simulink model "aaaqi"  (R2016b)
settings: Solver=ode4  StartTime=0.0  StopTime=inf  FixedStep=0.002  RelTol=1e-3  EnableMultiTasking=on
undefined symbols (not defined in the file or in its folder): bit, mdaadlink6208, sigbuilder_block, Standard
libraries: slrtlib x20, slrtsoftinglib x11, simulink x10
(part 2 of 4)

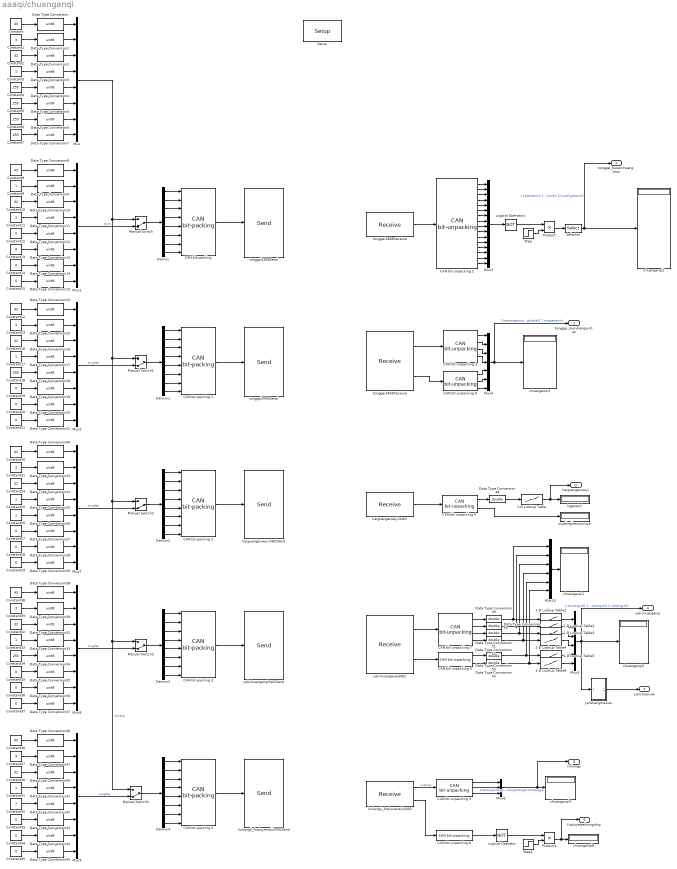
== system aaaqi/chuanganqi ==
  1-D Lookup Table : Lookup_n-D  NumberOfTableDimensions=1  BreakpointsForDimension1=[80 8500]  Table=[0 600]  InternalRulePriority=Speed  RndMeth=Simplest  InputSameDT=on
  1-D Lookup Table1 : Lookup_n-D  NumberOfTableDimensions=1  BreakpointsForDimension1=[1022 6022]  Table=[0 0.5]  InternalRulePriority=Speed  RndMeth=Simplest  InputSameDT=on
  1-D Lookup Table2 : Lookup_n-D  NumberOfTableDimensions=1  BreakpointsForDimension1=[1024 6018]  Table=[0 0.5]  InternalRulePriority=Speed  RndMeth=Simplest  InputSameDT=on
  1-D Lookup Table3 : Lookup_n-D  NumberOfTableDimensions=1  BreakpointsForDimension1=[999 5991]  Table=[0 0.5]  InternalRulePriority=Speed  RndMeth=Simplest  InputSameDT=on
  1-D Lookup Table4 : Lookup_n-D  NumberOfTableDimensions=1  BreakpointsForDimension1=[1006 6005]  Table=[0 0.5]  InternalRulePriority=Speed  RndMeth=Simplest  InputSameDT=on
  1-D Lookup Table5 : Lookup_n-D  NumberOfTableDimensions=1  BreakpointsForDimension1=[1010 6012]  Table=[0 0.5]  InternalRulePriority=Speed  RndMeth=Simplest  InputSameDT=on
  1-D Lookup Table6 : Lookup_n-D  NumberOfTableDimensions=1  BreakpointsForDimension1=[1024 6020]  Table=[0 0.5]  InternalRulePriority=Speed  RndMeth=Simplest  InputSameDT=on
  CAN bit-packing {,1..4} (5 alike) : slrtlib/CAN/Utilities/CAN bit-packing   bitpatterns={ [0:7] [8:15] [16:23] [24:31] [32:39] [40:47] [48:55] [56:63]}
  CAN bit-unpacking 2 : slrtlib/CAN/Utilities/CAN bit-unpacking   bitpatterns={0 1 2 3 4 5 6 7 8 9 10 11 12 13 14 15}  dtypes={ 'boolean','boolean','boolean','boolean','boolean','boolean','boolean','boolean','boolean','boolean','boolean','boolean','boolean','boolean','boolean','boolean'}
  CAN bit-unpacking 3 : slrtlib/CAN/Utilities/CAN bit-unpacking   bitpatterns={ [0:15],[16:31],[32:47],[48:63]}  dtypes={ 'uint16','uint16','uint16','uint16' }
  CAN bit-unpacking 4 : slrtlib/CAN/Utilities/CAN bit-unpacking   bitpatterns={ [0:15],[16:31]}  dtypes={ 'uint16','uint16'}
  CAN bit-unpacking 5 : slrtlib/CAN/Utilities/CAN bit-unpacking   bitpatterns={ [0:15] [16:31] [32:47]}  dtypes={ 'uint16','uint16','uint16'}
  CAN bit-unpacking 6 : slrtlib/CAN/Utilities/CAN bit-unpacking   bitpatterns={ [0:15],[16:31]}  dtypes={'uint16','uint16' }
  CAN bit-unpacking 7 : slrtlib/CAN/Utilities/CAN bit-unpacking   bitpatterns={ [0:15],[16:31],[32:47],[48:63]}  dtypes={ 'uint16','uint16','uint16','uint16' }
  CAN bit-unpacking 8 : slrtlib/CAN/Utilities/CAN bit-unpacking   bitpatterns={0}  dtypes={ 'boolean'}
  CAN bit-unpacking 9 : slrtlib/CAN/Utilities/CAN bit-unpacking   bitpatterns={ [0:15],[16:31],[32:47]}  dtypes={'uint16','uint16','uint16' }
  Constant{,8,22,30,38,46} (6 alike) : Constant  Value=43
  Constant{1,23,31,39,47} (5 alike) : Constant  Value=3
  Constant{2,10,16,24,32,40} (6 alike) : Constant  Value=32
  Constant{3,9,11,17,25..26,33,41} (8 alike) : Constant
  Constant{12..15,19..21,27..29,35..37,43..45} (16 alike) : Constant  Value=0
  Constant{4..7,18,34} (6 alike) : Constant  Value=255
  Constant42 : Constant  Value=7
  Data Type Conversion{,1..47} (48 alike) : DataTypeConversion  OutDataTypeStr=uint8
  Data Type Conversion{48..54} (7 alike) : DataTypeConversion  OutDataTypeStr=double
  Demux{,1..4} (5 alike) : Demux  Outputs=8
  Logical Operator : Logic  Operator=NOT  AllPortsSameDT=off  OutDataTypeStr=boolean
  Logical Operator1 : Logic  Operator=NOT  AllPortsSameDT=off  OutDataTypeStr=boolean
  Manual Switch{,1..4} (5 alike) : ManualSwitch  CurrentSetting=0
  Mux{,1..2,7..9} (6 alike) : Mux  Inputs=8
  Mux10 : Mux  Inputs=6
  Mux3 : Mux  Inputs=16
  Mux4 : Mux  Inputs=7
  Mux5 : Mux  Inputs=6
  Mux6 : Mux  Inputs=3
  Product : Product
  Product1 : Product
  Selector : Selector  IndexOptions=Index vector (dialog)  Indices=[5:16]  OutputSizes=[(-2)]
  "Setup " : slrtsoftinglib/CAN-AC2-PCI SJA 1000/Setup   board=1  can1bus=Highspeed (ISO 11898)  can1Baudrate=1 MBaud  can1UserBR=[1,1,4,3]  can2bus=Highspeed (ISO 11898)  can2Baudrate=500 kBaud  can2UserBR=[1,1,4,3]  init=[]  term=[]  bus_off_out=off  bus_off_rec=Off  ioBaseAddress=-1
  Step : Step  Time=0.2  SampleTime=0
  Step1 : Step  Time=0.2  SampleTime=0
  chuanganqi{1..5,8} (6 alike) : Display
  kaiguangaiweiyi3402 : slrtsoftinglib/CAN-AC2-PCI SJA 1000/Receive   board=1  canPort=CAN 1  range=Standard (11-bit)  ids=387  lengths=8  output=Data  inten=off  ts=-1  ididx=[2]
  kaiguangaiweiyi3402Send : slrtsoftinglib/CAN-AC2-PCI SJA 1000/Send   board=1  canPort=CAN 2  range=Standard (11-bit)  ids=1539  sizes=[8]  output=off  ts=-1  ididx=[1]
  kggweiyi : Display
  liuliangji_fuqiuyeweiji3402 : slrtsoftinglib/CAN-AC2-PCI SJA 1000/Receive   board=1  canPort=CAN 1  range=Standard (11-bit)  ids=[389 1157]  lengths=8  output=Data  inten=off  ts=-1  ididx=[4,7]
  liuliangji_fuqiuyeweiji3402Send : slrtsoftinglib/CAN-AC2-PCI SJA 1000/Send   board=1  canPort=CAN 2  range=Standard (11-bit)  ids=1541  sizes=[8]  output=off  ts=-1  ididx=[3]
  suodingjiesuoyouya : Display
  tonggai1808Receive : slrtsoftinglib/CAN-AC2-PCI SJA 1000/Receive   board=1  canPort=CAN 1  range=Standard (11-bit)  ids=385  lengths=8  output=Data  inten=off  ts=-1  ididx=[0]
  tonggai1808Send : slrtsoftinglib/CAN-AC2-PCI SJA 1000/Send   board=1  canPort=CAN 1  range=Standard (11-bit)  ids=1537  sizes=[8]  output=off  ts=-1  ididx=[0]
  tonggai3402Receive : slrtsoftinglib/CAN-AC2-PCI SJA 1000/Receive   board=1  canPort=CAN 1  range=Standard (11-bit)  ids=[386 642]  lengths=8  output=Data  inten=off  ts=-1  ididx=[1,5]
  tonggai3402Send : slrtsoftinglib/CAN-AC2-PCI SJA 1000/Send   board=1  canPort=CAN 2  range=Standard (11-bit)  ids=1538  sizes=[8]  output=off  ts=-1  ididx=[0]
  yalichuanganqi3402 : slrtsoftinglib/CAN-AC2-PCI SJA 1000/Receive   board=1  canPort=CAN 1  range=Standard (11-bit)  ids=[388 644]  lengths=8  output=Data  inten=off  ts=-1  ididx=[3,6]
  yalichuanganqi3402Send : slrtsoftinglib/CAN-AC2-PCI SJA 1000/Send   board=1  canPort=CAN 2  range=Standard (11-bit)  ids=1540  sizes=[8]  output=off  ts=-1  ididx=[2]
  yalishangxiaxian : Subsystem
  tonggai_huoerchuanganqi : Outport
  tonggai_moniliangxinhao : Outport  Port=2
  kaiguangaiweiyi : Outport  Port=3
  yalichuanganqi : Outport  Port=4
  liuliangji : Outport  Port=5
  fuqiuyeweikongzhiqi : Outport  Port=6
  yalichaoxian : Outport  Port=7
  wires:
  CAN bit-unpacking 3/1 -> Mux4/1
  CAN bit-unpacking 3/2 -> Mux4/2
  CAN bit-unpacking 3/3 -> Mux4/3
  CAN bit-unpacking 3/4 -> Mux4/4
  CAN bit-unpacking 4/1 -> Data Type Conversion48/1
  Mux3/1 -> Logical Operator1/1
  Mux4/1 -> tonggai_moniliangxinhao/1, chuanganqi3/1  "1.kaiguangaiyouya1 2.kaiguangaiyouya2 3.xuansongjinweiyi1 4.xuansongjinweiyi2 5.xuansongjinlayali1 6.xuansongjinlayali2 7.tonggaijiasudu"
  kaiguangaiweiyi3402/1 -> CAN bit-unpacking 4/1
  tonggai3402Receive/1 -> CAN bit-unpacking 3/1
  tonggai1808Receive/1 -> CAN bit-unpacking 2/1
  Data Type Conversion/1 -> Mux/1
  Data Type Conversion1/1 -> Mux/2
  Data Type Conversion2/1 -> Mux/3
  Data Type Conversion3/1 -> Mux/4
  Data Type Conversion4/1 -> Mux/5
  Data Type Conversion5/1 -> Mux/6
  Data Type Conversion6/1 -> Mux/7
  Data Type Conversion7/1 -> Mux/8
  Demux/1 -> "CAN bit-packing "/1
  Demux/2 -> "CAN bit-packing "/2
  Demux/3 -> "CAN bit-packing "/3
  Demux/4 -> "CAN bit-packing "/4
  Demux/5 -> "CAN bit-packing "/5
  Demux/6 -> "CAN bit-packing "/6
  Demux/7 -> "CAN bit-packing "/7
  Demux/8 -> "CAN bit-packing "/8
  "CAN bit-packing "/1 -> tonggai1808Send/1
  Constant/1 -> Data Type Conversion/1
  Constant1/1 -> Data Type Conversion1/1
  Constant2/1 -> Data Type Conversion2/1
  Constant3/1 -> Data Type Conversion3/1
  Constant4/1 -> Data Type Conversion4/1
  Constant5/1 -> Data Type Conversion5/1
  Constant6/1 -> Data Type Conversion6/1
  Constant7/1 -> Data Type Conversion7/1
  Demux1/1 -> CAN bit-packing 1/1
  Demux1/2 -> CAN bit-packing 1/2
  Demux1/3 -> CAN bit-packing 1/3
  Demux1/4 -> CAN bit-packing 1/4
  Demux1/5 -> CAN bit-packing 1/5
  Demux1/6 -> CAN bit-packing 1/6
  Demux1/7 -> CAN bit-packing 1/7
  Demux1/8 -> CAN bit-packing 1/8
  CAN bit-packing 1/1 -> tonggai3402Send/1
  Demux2/1 -> CAN bit-packing 2/1
  Demux2/2 -> CAN bit-packing 2/2
  Demux2/3 -> CAN bit-packing 2/3
  Demux2/4 -> CAN bit-packing 2/4
  Demux2/5 -> CAN bit-packing 2/5
  Demux2/6 -> CAN bit-packing 2/6
  Demux2/7 -> CAN bit-packing 2/7
  Demux2/8 -> CAN bit-packing 2/8
  CAN bit-packing 2/1 -> kaiguangaiweiyi3402Send/1
  Data Type Conversion8/1 -> Mux1/1
  Data Type Conversion9/1 -> Mux1/2
  Data Type Conversion10/1 -> Mux1/3
  Data Type Conversion11/1 -> Mux1/4
  Data Type Conversion12/1 -> Mux1/5
  Data Type Conversion13/1 -> Mux1/6
  Data Type Conversion14/1 -> Mux1/7
  Data Type Conversion15/1 -> Mux1/8
  Constant8/1 -> Data Type Conversion8/1
  Constant9/1 -> Data Type Conversion9/1
  Constant10/1 -> Data Type Conversion10/1
  Constant11/1 -> Data Type Conversion11/1
  Constant12/1 -> Data Type Conversion12/1
  Constant13/1 -> Data Type Conversion13/1
  Constant14/1 -> Data Type Conversion14/1
  Constant15/1 -> Data Type Conversion15/1
  Data Type Conversion22/1 -> Mux2/1
  Data Type Conversion23/1 -> Mux2/2
  Data Type Conversion16/1 -> Mux2/3
  Data Type Conversion17/1 -> Mux2/4
  Data Type Conversion18/1 -> Mux2/5
  Data Type Conversion19/1 -> Mux2/6
  Data Type Conversion20/1 -> Mux2/7
  Data Type Conversion21/1 -> Mux2/8
  Constant22/1 -> Data Type Conversion22/1
  Constant23/1 -> Data Type Conversion23/1
  Constant16/1 -> Data Type Conversion16/1
  Constant17/1 -> Data Type Conversion17/1
  Constant18/1 -> Data Type Conversion18/1
  Constant19/1 -> Data Type Conversion19/1
  Constant20/1 -> Data Type Conversion20/1
  Constant21/1 -> Data Type Conversion21/1
  Data Type Conversion30/1 -> Mux7/1
  Data Type Conversion31/1 -> Mux7/2
  Data Type Conversion24/1 -> Mux7/3
  Data Type Conversion25/1 -> Mux7/4
  Data Type Conversion26/1 -> Mux7/5
  Data Type Conversion27/1 -> Mux7/6
  Data Type Conversion28/1 -> Mux7/7
  Data Type Conversion29/1 -> Mux7/8
  Constant30/1 -> Data Type Conversion30/1
  Constant31/1 -> Data Type Conversion31/1
  Constant24/1 -> Data Type Conversion24/1
  Constant25/1 -> Data Type Conversion25/1
  Constant26/1 -> Data Type Conversion26/1
  Constant27/1 -> Data Type Conversion27/1
  Constant28/1 -> Data Type Conversion28/1
  Constant29/1 -> Data Type Conversion29/1
  Manual Switch/1 -> Demux/1
  Manual Switch1/1 -> Demux1/1
  Manual Switch2/1 -> Demux2/1
  Mux7/1 -> Manual Switch2/2  "tongdao"
  Mux2/1 -> Manual Switch1/2  "tongdao"
  Mux1/1 -> Manual Switch/2  "shuru"
  Mux/1 -> Manual Switch1/1, Manual Switch2/1, Manual Switch3/1, Manual Switch4/1, Manual Switch/1  "shineng"
  CAN bit-unpacking 2/1 -> Mux3/1
  CAN bit-unpacking 2/2 -> Mux3/2
  CAN bit-unpacking 2/3 -> Mux3/3
  CAN bit-unpacking 2/4 -> Mux3/4
  CAN bit-unpacking 2/5 -> Mux3/5
  CAN bit-unpacking 2/6 -> Mux3/6
  CAN bit-unpacking 2/7 -> Mux3/7
  CAN bit-unpacking 2/8 -> Mux3/8
  CAN bit-unpacking 2/9 -> Mux3/9
  CAN bit-unpacking 2/10 -> Mux3/10
  CAN bit-unpacking 2/11 -> Mux3/11
  CAN bit-unpacking 2/12 -> Mux3/12
  CAN bit-unpacking 2/13 -> Mux3/13
  CAN bit-unpacking 2/14 -> Mux3/14
  CAN bit-unpacking 2/15 -> Mux3/15
  CAN bit-unpacking 2/16 -> Mux3/16
  tonggai3402Receive/2 -> CAN bit-unpacking 9/1
  CAN bit-unpacking 9/1 -> Mux4/5
  CAN bit-unpacking 9/2 -> Mux4/6
  yalichuanganqi3402/1 -> CAN bit-unpacking 7/1
  yalichuanganqi3402/2 -> CAN bit-unpacking 6/1
  liuliangji_fuqiuyeweiji3402/1 -> CAN bit-unpacking 5/1  "liuliangji"
  CAN bit-unpacking 5/1 -> Mux6/1
  CAN bit-unpacking 5/2 -> Mux6/2
  CAN bit-unpacking 5/3 -> Mux6/3
  Mux6/1 -> liuliangji/1, chuanganqi4/1  "1.liantongliuliangji1 2.liandongliuliangji2 3.liuliangji3"
  Mux5/1 -> yalichuanganqi/1, chuanganqi5/1, yalishangxiaxian/1(In1)  "1.shuicangyali1 2.shuicangyali2 3.shangqiangyali1 4.shangqiangyali2 5.xiaqiangyali1 6.xiaqiangyali2"
  Demux3/1 -> CAN bit-packing 3/1
  Demux3/2 -> CAN bit-packing 3/2
  Demux3/3 -> CAN bit-packing 3/3
  Demux3/4 -> CAN bit-packing 3/4
  Demux3/5 -> CAN bit-packing 3/5
  Demux3/6 -> CAN bit-packing 3/6
  Demux3/7 -> CAN bit-packing 3/7
  Demux3/8 -> CAN bit-packing 3/8
  CAN bit-packing 3/1 -> yalichuanganqi3402Send/1
  Demux4/1 -> CAN bit-packing 4/1
  Demux4/2 -> CAN bit-packing 4/2
  Demux4/3 -> CAN bit-packing 4/3
  Demux4/4 -> CAN bit-packing 4/4
  Demux4/5 -> CAN bit-packing 4/5
  Demux4/6 -> CAN bit-packing 4/6
  Demux4/7 -> CAN bit-packing 4/7
  Demux4/8 -> CAN bit-packing 4/8
  CAN bit-packing 4/1 -> liuliangji_fuqiuyeweiji3402Send/1
  Data Type Conversion38/1 -> Mux8/1
  Data Type Conversion39/1 -> Mux8/2
  Data Type Conversion32/1 -> Mux8/3
  Data Type Conversion33/1 -> Mux8/4
  Data Type Conversion34/1 -> Mux8/5
  Data Type Conversion35/1 -> Mux8/6
  Data Type Conversion36/1 -> Mux8/7
  Data Type Conversion37/1 -> Mux8/8
  Constant38/1 -> Data Type Conversion38/1
  Constant39/1 -> Data Type Conversion39/1
  Constant32/1 -> Data Type Conversion32/1
  Constant33/1 -> Data Type Conversion33/1
  Constant34/1 -> Data Type Conversion34/1
  Constant35/1 -> Data Type Conversion35/1
  Constant36/1 -> Data Type Conversion36/1
  Constant37/1 -> Data Type Conversion37/1
  Data Type Conversion46/1 -> Mux9/1
  Data Type Conversion47/1 -> Mux9/2
  Data Type Conversion40/1 -> Mux9/3
  Data Type Conversion41/1 -> Mux9/4
  Data Type Conversion42/1 -> Mux9/5
  Data Type Conversion43/1 -> Mux9/6
  Data Type Conversion44/1 -> Mux9/7
  Data Type Conversion45/1 -> Mux9/8
  Constant46/1 -> Data Type Conversion46/1
  Constant47/1 -> Data Type Conversion47/1
  Constant40/1 -> Data Type Conversion40/1
  Constant41/1 -> Data Type Conversion41/1
  Constant42/1 -> Data Type Conversion42/1
  Constant43/1 -> Data Type Conversion43/1
  Constant44/1 -> Data Type Conversion44/1
  Constant45/1 -> Data Type Conversion45/1
  Manual Switch3/1 -> Demux3/1
  Mux8/1 -> Manual Switch3/2  "tongdao"
  Mux9/1 -> Manual Switch4/2  "tongdao"
  Manual Switch4/1 -> Demux4/1
  CAN bit-unpacking 8/1 -> Logical Operator/1
  Step/1 -> Product/2
  Logical Operator1/1 -> Product/1
  Product/1 -> Selector/1
  Step1/1 -> Product1/2
  Logical Operator/1 -> Product1/1
  Product1/1 -> fuqiuyeweikongzhiqi/1, chuanganqi8/1
  liuliangji_fuqiuyeweiji3402/2 -> CAN bit-unpacking 8/1
  CAN bit-unpacking 4/2 -> suodingjiesuoyouya/1
  yalishangxiaxian/1(Out1) -> yalichaoxian/1
  CAN bit-unpacking 9/3 -> Mux4/7
  1-D Lookup Table/1 -> kaiguangaiweiyi/1, kggweiyi/1
  Data Type Conversion48/1 -> 1-D Lookup Table/1
  Data Type Conversion49/1 -> 1-D Lookup Table1/1, Mux10/1
  Data Type Conversion50/1 -> 1-D Lookup Table2/1, Mux10/2
  Data Type Conversion51/1 -> 1-D Lookup Table3/1, Mux10/3
  Data Type Conversion52/1 -> 1-D Lookup Table4/1, Mux10/4
  Data Type Conversion53/1 -> 1-D Lookup Table5/1, Mux10/5
  Data Type Conversion54/1 -> 1-D Lookup Table6/1, Mux10/6
  CAN bit-unpacking 6/2 -> Data Type Conversion54/1
  CAN bit-unpacking 7/1 -> Data Type Conversion49/1
  CAN bit-unpacking 7/2 -> Data Type Conversion50/1
  CAN bit-unpacking 7/3 -> Data Type Conversion51/1
  CAN bit-unpacking 7/4 -> Data Type Conversion52/1
  CAN bit-unpacking 6/1 -> Data Type Conversion53/1
  1-D Lookup Table1/1 -> Mux5/1
  1-D Lookup Table2/1 -> Mux5/2
  1-D Lookup Table3/1 -> Mux5/3
  1-D Lookup Table4/1 -> Mux5/4
  1-D Lookup Table5/1 -> Mux5/5
  1-D Lookup Table6/1 -> Mux5/6
  Mux10/1 -> chuanganqi1/1
  Selector/1 -> tonggai_huoerchuanganqi/1, chuanganqi2/1  "1.kaigaidaowei 2.kaigaihuanchong 3.guangaidaowei 4.guangaihuanchong 5.xuanjindaowei1 6.xuanjindaowei2 7.xuansongdaowei1 8.xuansongdaowei2 9.jiesuodaowei1 10.jiesuodaowei2 11.suodingdaowei1 12.suodingdaowei2"

== system aaaqi/guangaiquxian ==
  In1 : Inport
  In2 : Inport  Port=2
  Add : Sum
  Chart1 : Stateflow chart  TreatAsAtomicUnit=on
  Display : Display
  Fcn : Fcn  Expr=(3.76012963313985e-12)*u^16-(3.44037229998304e-10)*u^15+(1.39996774652558e-08)*u^14-(3.34309394387153e-07)*u^13+(5.21860519506510e-06)*u^12-(5.63398801585665e-05)*u^11+0.000435175092700704*u^10-0.00244274561068785*u^9+0.00982136561852038*u^8-0.0269377658736148*u^7+0.0514170009108526*u^6-0.103245210636221*u^5+0.431283025667506*u^4-2.79148222601809*u^3+0.0172306812740196*u^2-0.00241932536131526*u+600.000082443648
  Saturation : Saturate  UpperLimit=12  LowerLimit=0
  Saturation1 : Saturate  UpperLimit=600  LowerLimit=20
  Out1 : Outport
  wires:
  In1/1 -> Chart1/1(a)
  Chart1/1(t) -> Saturation/1
  Saturation/1 -> Fcn/1
  Fcn/1 -> Saturation1/1
  Add/1 -> Out1/1, Display/1
  Saturation1/1 -> Add/1
  In2/1 -> Add/2

== system aaaqi/jinjichuli ==
  tiaoshi : Inport
  fa : Inport  Port=2
  jiting : Inport  Port=3
  Enable : EnablePort  StatesWhenEnabling=reset
  Demux : Demux  Outputs=16
  Mux : Mux  Inputs=16
  jinjichuli : Stateflow chart  TreatAsAtomicUnit=on
  Out1 : Outport
  wires:
  tiaoshi/1 -> jinjichuli/1(tiaoshi)
  fa/1 -> Demux/1
  Demux/1 -> jinjichuli/2(fa11_1)
  Demux/2 -> jinjichuli/3(fa11_2)
  Demux/3 -> jinjichuli/4(fa11_5)
  Demux/4 -> jinjichuli/5(fa20)
  Demux/5 -> jinjichuli/6(fa16_1)
  Demux/6 -> jinjichuli/7(fa3)
  Demux/7 -> jinjichuli/8(fa21)
  Demux/12 -> jinjichuli/13(fa18_1)
  Demux/13 -> jinjichuli/14(fa18_2)
  jiting/1 -> jinjichuli/18(jiting)
  Demux/14 -> jinjichuli/15(fa18_3)
  Demux/15 -> jinjichuli/16(fa18_4)
  Demux/16 -> jinjichuli/17(fa_kgg)
  jinjichuli/1(diancifa11_1) -> Mux/1
  jinjichuli/2(diancifa11_2) -> Mux/2
  jinjichuli/3(diancifa11_5) -> Mux/3
  jinjichuli/4(diancifa20) -> Mux/4
  jinjichuli/5(diancifa16_1) -> Mux/5
  jinjichuli/6(diancifa3) -> Mux/6
  jinjichuli/7(diancifa21) -> Mux/7
  jinjichuli/12(bililiuliangfa18_1) -> Mux/12
  jinjichuli/13(bililiuliangfa18_2) -> Mux/13
  jinjichuli/14(bililiuliangfa18_3) -> Mux/14
  jinjichuli/15(bililiuliangfa18_4) -> Mux/15
  jinjichuli/16(kaiguangaifa) -> Mux/16
  Mux/1 -> Out1/1
  Demux/8 -> jinjichuli/9(suodingmingling)
  Demux/9 -> jinjichuli/10(jiesuomingling)
  Demux/10 -> jinjichuli/11(xuansongmingling)
  Demux/11 -> jinjichuli/12(xuanjinmingling)
  jinjichuli/8(suoding) -> Mux/8
  jinjichuli/9(jiesuo) -> Mux/9
  jinjichuli/10(xuansong) -> Mux/10
  jinjichuli/11(xuanjin) -> Mux/11

== system aaaqi/kaigaiquxian ==
  In1 : Inport
  In2 : Inport  Port=2
  Add : Sum
  Chart : Stateflow chart  TreatAsAtomicUnit=on
  Display : Display
  Fcn : Fcn  Expr=(3.76012794303783e-12)*u^16-(3.77787151438439e-10)*u^15+(1.70366716702520e-08)*u^14-(4.53918294904343e-07)*u^13+(7.91595568148143e-06)*u^12-(9.46991801150381e-05)*u^11+0.000795158956924619*u^10-0.00475883386986616*u^9+0.0207391801532158*u^8-0.0673081776269616*u^7+0.155366359479885*u^6-0.201490925155371*u^5-0.0768516231318135*u^4+2.18034933328387*u^3+0.0584293012534094*u^2-0.00654372848246011*u+20.0002376678902
  Saturation : Saturate  UpperLimit=12  LowerLimit=0
  Saturation1 : Saturate  UpperLimit=600  LowerLimit=20
  Out1 : Outport
  wires:
  In1/1 -> Chart/1(a)
  Saturation/1 -> Fcn/1
  Chart/1(t) -> Saturation/1
  Fcn/1 -> Saturation1/1
  Add/1 -> Display/1, Out1/1
  Saturation1/1 -> Add/1
  In2/1 -> Add/2

== system aaaqi/tiaoshifa ==
  Mux3 : Mux  Inputs=16
  fa11_1 : Constant  Value=0
      settings: OpenFcn=|
      | if get_param(gcb,'value')=='1',
      | set_param(gcb,'value','0');
      | else
      | set_param(gcb,'value','1');end
  fa11_2 : Constant  Value=0
      settings: OpenFcn=|
      | if get_param(gcb,'value')=='1',
      | set_param(gcb,'value','0');
      | else
      | set_param(gcb,'value','1');end
  fa11_5 : Constant  Value=0
      settings: OpenFcn=|
      | if get_param(gcb,'value')=='1',
      | set_param(gcb,'value','0');
      | else
      | set_param(gcb,'value','1');end
  fa16_1 : Constant  Value=0
      settings: OpenFcn=|
      | if get_param(gcb,'value')=='1',
      | set_param(gcb,'value','0');
      | else
      | set_param(gcb,'value','1');end
  fa18_{1..4} (4 alike) : Constant  Value=0
  fa20 : Constant  Value=0
      settings: OpenFcn=|
      | if get_param(gcb,'value')=='1',
      | set_param(gcb,'value','0');
      | else
      | set_param(gcb,'value','1');end
  fa21 : Constant  Value=0
      settings: OpenFcn=|
      | if get_param(gcb,'value')=='1',
      | set_param(gcb,'value','0');
      | else
      | set_param(gcb,'value','1');end
  fa3 : Constant  Value=0
      settings: OpenFcn=|
      | if get_param(gcb,'value')=='1',
      | set_param(gcb,'value','0');
      | else
      | set_param(gcb,'value','1');end
  fa_kgg : Constant  Value=0
  jiesuomingling : Constant  Value=0
      settings: OpenFcn=|
      | if get_param(gcb,'value')=='1',
      | set_param(gcb,'value','0');
      | else
      | set_param(gcb,'value','1');end
  suodingmingling : Constant  Value=0
      settings: OpenFcn=|
      | if get_param(gcb,'value')=='1',
      | set_param(gcb,'value','0');
      | else
      | set_param(gcb,'value','1');end
  xuanjinmingling : Constant  Value=0
      settings: OpenFcn=|
      | if get_param(gcb,'value')=='1',
      | set_param(gcb,'value','0');
      | else
      | set_param(gcb,'value','1');end
  xuansongmingling : Constant  Value=0
      settings: OpenFcn=|
      | if get_param(gcb,'value')=='1',
      | set_param(gcb,'value','0');
      | else
      | set_param(gcb,'value','1');end
  Out1 : Outport
  wires:
  fa11_5/1 -> Mux3/3
  fa20/1 -> Mux3/4
  jiesuomingling/1 -> Mux3/11
  xuanjinmingling/1 -> Mux3/9
  fa_kgg/1 -> Mux3/16
  fa11_2/1 -> Mux3/2
  fa11_1/1 -> Mux3/1
  fa16_1/1 -> Mux3/5
  xuansongmingling/1 -> Mux3/8
  fa21/1 -> Mux3/7
  suodingmingling/1 -> Mux3/10
  fa3/1 -> Mux3/6
  Mux3/1 -> Out1/1
  fa18_1/1 -> Mux3/12
  fa18_2/1 -> Mux3/13
  fa18_3/1 -> Mux3/14
  fa18_4/1 -> Mux3/15

== system aaaqi/Subsystem2/husuo ==
  In1 : Inport
  In2 : Inport  Port=2
  Constant : Constant  Value=0
  Constant2 : Constant  Value=0
  Memory : Memory
  Memory1 : Memory
  Switch : Switch  Criteria=u2 > Threshold  Threshold=0.5
  Switch2 : Switch  Criteria=u2 > Threshold  Threshold=0.5
  Out1 : Outport
  Out2 : Outport  Port=2
  wires:
  Memory/1 -> Switch/2
  Memory1/1 -> Switch2/2
  In1/1 -> Switch/3
  In2/1 -> Switch2/3
  Constant2/1 -> Switch2/1
  Switch/1 -> Memory1/1, Out1/1
  Constant/1 -> Switch/1
  Switch2/1 -> Out2/1, Memory/1

== system aaaqi/Subsystem2/husuo1 ==
  In1 : Inport
  In2 : Inport  Port=2
  Constant : Constant  Value=0
  Constant2 : Constant  Value=0
  Memory : Memory
  Memory1 : Memory
  Switch : Switch  Criteria=u2 > Threshold  Threshold=0.5
  Switch2 : Switch  Criteria=u2 > Threshold  Threshold=0.5
  Out1 : Outport
  Out2 : Outport  Port=2
  wires:
  Switch2/1 -> Memory/1, Out2/1
  Constant/1 -> Switch/1
  Switch/1 -> Out1/1, Memory1/1
  Constant2/1 -> Switch2/1
  In2/1 -> Switch2/3
  In1/1 -> Switch/3
  Memory1/1 -> Switch2/2
  Memory/1 -> Switch/2

== system aaaqi/Subsystem2/husuo2 ==
  In1 : Inport
  In2 : Inport  Port=2
  Constant : Constant  Value=0
  Constant2 : Constant  Value=0
  Memory : Memory
  Memory1 : Memory
  Switch : Switch  Criteria=u2 > Threshold  Threshold=0.5
  Switch2 : Switch  Criteria=u2 > Threshold  Threshold=0.5
  Out1 : Outport
  Out2 : Outport  Port=2
  wires:
  Memory/1 -> Switch/2
  Memory1/1 -> Switch2/2
  In1/1 -> Switch/3
  In2/1 -> Switch2/3
  Constant2/1 -> Switch2/1
  Switch/1 -> Memory1/1, Out1/1
  Constant/1 -> Switch/1
  Switch2/1 -> Out2/1, Memory/1

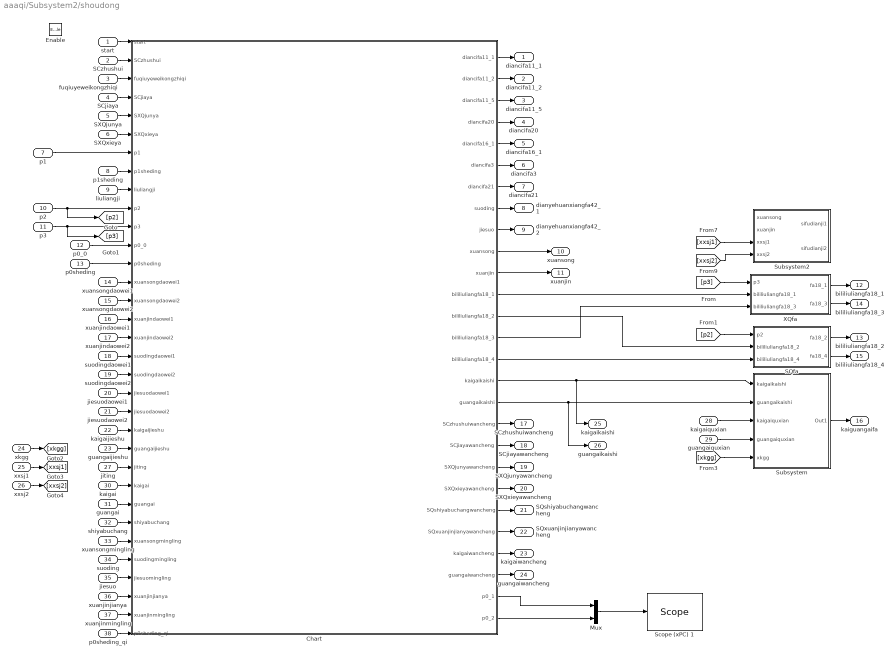
== system aaaqi/Subsystem2/shoudong ==
  start : Inport
  SCzhushui : Inport  Port=2
  fuqiuyeweikongzhiqi : Inport  Port=3
  SCjiaya : Inport  Port=4
  SXQjunya : Inport  Port=5
  SXQxieya : Inport  Port=6
  p1 : Inport  Port=7
  p1sheding : Inport  Port=8
  liuliangji : Inport  Port=9
  p2 : Inport  Port=10
  p3 : Inport  Port=11
  p0_0 : Inport  Port=12
  p0sheding : Inport  Port=13
  xuansongdaowei1 : Inport  Port=14
  xuansongdaowei2 : Inport  Port=15
  xuanjindaowei1 : Inport  Port=16
  xuanjindaowei2 : Inport  Port=17
  suodingdaowei1 : Inport  Port=18
  suodingdaowei2 : Inport  Port=19
  jiesuodaowei1 : Inport  Port=20
  jiesuodaowei2 : Inport  Port=21
  kaigaijieshu : Inport  Port=22
  guangaijieshu : Inport  Port=23
  xkgg : Inport  Port=24
  xxsj1 : Inport  Port=25
  xxsj2 : Inport  Port=26
  jiting : Inport  Port=27
  kaigaiquxian : Inport  Port=28
  guangaiquxian : Inport  Port=29
  kaigai : Inport  Port=30
  guangai : Inport  Port=31
  shiyabuchang : Inport  Port=32
  xuansongmingling : Inport  Port=33
  suoding : Inport  Port=34
  jiesuo : Inport  Port=35
  xuanjinjianya : Inport  Port=36
  xuanjinmingling : Inport  Port=37
  p0sheding_qi : Inport  Port=38
  Enable : EnablePort
  Chart : Stateflow chart  TreatAsAtomicUnit=on
  Mux : Mux  Inputs=2
  SQfa : Subsystem
  Scope (xPC) 1 : slrtlib/Displays and Logging/Scope   scopeno=5  scopetype=Target  autostart=on  viewmode=Numerical  formatstr='%15.6f'  grid=on  ylimits=[0,0]  nosamples=250  noprepostsamples=0  interleave=1  triggermode=FreeRun  triggersignal=1  trigsignalfromport=off  triggerlevel=0.0  triggerslope=Either  triggerscope=1  triggersample=0  filename=data.dat  mode=Lazy  writesize=512  autorestart=off  dynamicfilemode=off  maxwritefilesize=512*1024^2
  Subsystem : Subsystem
  Subsystem2 : Subsystem
  XQfa : Subsystem
  diancifa11_1 : Outport
  diancifa11_2 : Outport  Port=2
  diancifa11_5 : Outport  Port=3
  diancifa20 : Outport  Port=4
  diancifa16_1 : Outport  Port=5
  diancifa3 : Outport  Port=6
  diancifa21 : Outport  Port=7
  dianyehuanxiangfa42_1 : Outport  Port=8
  dianyehuanxiangfa42_2 : Outport  Port=9
  xuansong : Outport  Port=10
  xuanjin : Outport  Port=11
  bililiuliangfa18_1 : Outport  Port=12
  bililiuliangfa18_2 : Outport  Port=13
  bililiuliangfa18_3 : Outport  Port=14
  bililiuliangfa18_4 : Outport  Port=15
  kaiguangaifa : Outport  Port=16
  SCzhushuiwancheng : Outport  Port=17
  SCjiayawancheng : Outport  Port=18
  SXQjunyawancheng : Outport  Port=19
  SXQxieyawancheng : Outport  Port=20
  SQshiyabuchangwancheng : Outport  Port=21
  SQxuanjinjianyawancheng : Outport  Port=22
  kaigaiwancheng : Outport  Port=23
  guangaiwancheng : Outport  Port=24
  kaigaikaishi : Outport  Port=25
  guangaikaishi : Outport  Port=26
  wires:
  jiting/1 -> Chart/24(jiting)
  xkgg/1 -> [xkgg]
  Chart/23(SQxuanjinjianyawancheng) -> SQxuanjinjianyawancheng/1
  Chart/22(SQshiyabuchangwancheng) -> SQshiyabuchangwancheng/1
  Chart/21(SXQxieyawancheng) -> SXQxieyawancheng/1
  Chart/20(SXQjunyawancheng) -> SXQjunyawancheng/1
  Chart/19(SCjiayawancheng) -> SCjiayawancheng/1
  Chart/18(SCzhushuiwancheng) -> SCzhushuiwancheng/1
  Chart/9(jiesuo) -> dianyehuanxiangfa42_2/1
  Chart/8(suoding) -> dianyehuanxiangfa42_1/1
  Chart/25(guangaiwancheng) -> guangaiwancheng/1
  guangaijieshu/1 -> Chart/23(guangaijieshu)
  Chart/24(kaigaiwancheng) -> kaigaiwancheng/1
  kaigaijieshu/1 -> Chart/22(kaigaijieshu)
  jiesuodaowei2/1 -> Chart/21(jiesuodaowei2)
  jiesuodaowei1/1 -> Chart/20(jiesuodaowei1)
  suodingdaowei2/1 -> Chart/19(suodingdaowei2)
  suodingdaowei1/1 -> Chart/18(suodingdaowei1)
  xuanjindaowei2/1 -> Chart/17(xuanjindaowei2)
  xuanjindaowei1/1 -> Chart/16(xuanjindaowei1)
  xuansongdaowei2/1 -> Chart/15(xuansongdaowei2)
  xuansongdaowei1/1 -> Chart/14(xuansongdaowei1)
  guangai/1 -> Chart/26(guangai)
  kaigai/1 -> Chart/25(kaigai)
  SQfa/2(fa18_4) -> bililiuliangfa18_4/1
  SQfa/1(fa18_2) -> bililiuliangfa18_2/1
  liuliangji/1 -> Chart/9(liuliangji)
  XQfa/2(fa18_3) -> bililiuliangfa18_3/1
  Chart/7(diancifa21) -> diancifa21/1
  XQfa/1(fa18_1) -> bililiuliangfa18_1/1
  Chart/6(diancifa3) -> diancifa3/1
  SXQxieya/1 -> Chart/6(SXQxieya)
  Chart/5(diancifa16_1) -> diancifa16_1/1
  SXQjunya/1 -> Chart/5(SXQjunya)
  Chart/4(diancifa20) -> diancifa20/1
  SCjiaya/1 -> Chart/4(SCjiaya)
  Chart/3(diancifa11_5) -> diancifa11_5/1
  fuqiuyeweikongzhiqi/1 -> Chart/3(fuqiuyeweikongzhiqi)
  Chart/2(diancifa11_2) -> diancifa11_2/1
  SCzhushui/1 -> Chart/2(SCzhushui)
  Chart/1(diancifa11_1) -> diancifa11_1/1
  start/1 -> Chart/1(start)
  p1/1 -> Chart/7(p1)
  [p2] -> SQfa/1(p2)
  [p3] -> XQfa/1(p3)
  p3/1 -> [p3], Chart/11(p3)
  p2/1 -> [p2], Chart/10(p2)
  p0_0/1 -> Chart/12(p0_0)
  p0sheding/1 -> Chart/13(p0sheding)
  p1sheding/1 -> Chart/8(p1sheding)
  Chart/15(bililiuliangfa18_4) -> SQfa/3(bililiuliangfa18_4)
  Chart/12(bililiuliangfa18_1) -> XQfa/2(bililiuliangfa18_1)
  Chart/13(bililiuliangfa18_2) -> SQfa/2(bililiuliangfa18_2)
  Chart/14(bililiuliangfa18_3) -> XQfa/3(bililiuliangfa18_3)
  shiyabuchang/1 -> Chart/27(shiyabuchang)
  xuansongmingling/1 -> Chart/28(xuansongmingling)
  suoding/1 -> Chart/29(suodingmingling)
  jiesuo/1 -> Chart/30(jiesuomingling)
  xuanjinjianya/1 -> Chart/31(xuanjinjianya)
  xuanjinmingling/1 -> Chart/32(xuanjinmingling)
  xxsj1/1 -> [xxsj1]
  xxsj2/1 -> [xxsj2]
  [xkgg] -> Subsystem/5(xkgg)
  Subsystem/1(Out1) -> kaiguangaifa/1
  [xxsj2] -> Subsystem2/4(xxsj2)
  [xxsj1] -> Subsystem2/3(xxsj1)
  Chart/10(xuansong) -> xuansong/1
  Chart/11(xuanjin) -> xuanjin/1
  Chart/26(p0_1) -> Mux/1
  Chart/27(p0_2) -> Mux/2
  Mux/1 -> Scope (xPC) 1/1
  Chart/16(kaigaikaishi) -> kaigaikaishi/1, Subsystem/1(kaigaikaishi)
  Chart/17(guangaikaishi) -> Subsystem/2(guangaikaishi), guangaikaishi/1
  guangaiquxian/1 -> Subsystem/4(guangaiquxian)
  kaigaiquxian/1 -> Subsystem/3(kaigaiquxian)
  p0sheding_qi/1 -> Chart/33(p0sheding_qi)

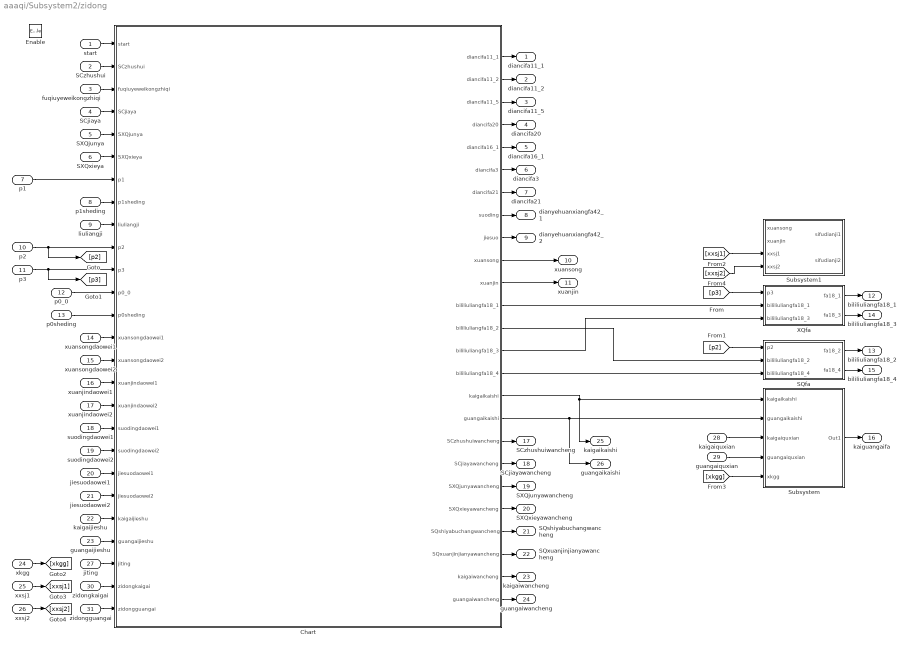
== system aaaqi/Subsystem2/zidong ==
  start : Inport
  SCzhushui : Inport  Port=2
  fuqiuyeweikongzhiqi : Inport  Port=3
  SCjiaya : Inport  Port=4
  SXQjunya : Inport  Port=5
  SXQxieya : Inport  Port=6
  p1 : Inport  Port=7
  p1sheding : Inport  Port=8
  liuliangji : Inport  Port=9
  p2 : Inport  Port=10
  p3 : Inport  Port=11
  p0_0 : Inport  Port=12
  p0sheding : Inport  Port=13
  xuansongdaowei1 : Inport  Port=14
  xuansongdaowei2 : Inport  Port=15
  xuanjindaowei1 : Inport  Port=16
  xuanjindaowei2 : Inport  Port=17
  suodingdaowei1 : Inport  Port=18
  suodingdaowei2 : Inport  Port=19
  jiesuodaowei1 : Inport  Port=20
  jiesuodaowei2 : Inport  Port=21
  kaigaijieshu : Inport  Port=22
  guangaijieshu : Inport  Port=23
  xkgg : Inport  Port=24
  xxsj1 : Inport  Port=25
  xxsj2 : Inport  Port=26
  jiting : Inport  Port=27
  kaigaiquxian : Inport  Port=28
  guangaiquxian : Inport  Port=29
  zidongkaigai : Inport  Port=30
  zidongguangai : Inport  Port=31
  Enable : EnablePort
  Chart : Stateflow chart  TreatAsAtomicUnit=on
  SQfa : Subsystem
  Subsystem : Subsystem
  Subsystem1 : Subsystem
  XQfa : Subsystem
  diancifa11_1 : Outport
  diancifa11_2 : Outport  Port=2
  diancifa11_5 : Outport  Port=3
  diancifa20 : Outport  Port=4
  diancifa16_1 : Outport  Port=5
  diancifa3 : Outport  Port=6
  diancifa21 : Outport  Port=7
  dianyehuanxiangfa42_1 : Outport  Port=8
  dianyehuanxiangfa42_2 : Outport  Port=9
  xuansong : Outport  Port=10
  xuanjin : Outport  Port=11
  bililiuliangfa18_1 : Outport  Port=12
  bililiuliangfa18_2 : Outport  Port=13
  bililiuliangfa18_3 : Outport  Port=14
  bililiuliangfa18_4 : Outport  Port=15
  kaiguangaifa : Outport  Port=16
  SCzhushuiwancheng : Outport  Port=17
  SCjiayawancheng : Outport  Port=18
  SXQjunyawancheng : Outport  Port=19
  SXQxieyawancheng : Outport  Port=20
  SQshiyabuchangwancheng : Outport  Port=21
  SQxuanjinjianyawancheng : Outport  Port=22
  kaigaiwancheng : Outport  Port=23
  guangaiwancheng : Outport  Port=24
  kaigaikaishi : Outport  Port=25
  guangaikaishi : Outport  Port=26
  wires:
  Chart/14(bililiuliangfa18_3) -> XQfa/3(bililiuliangfa18_3)
  Chart/13(bililiuliangfa18_2) -> SQfa/2(bililiuliangfa18_2)
  Chart/12(bililiuliangfa18_1) -> XQfa/2(bililiuliangfa18_1)
  Chart/15(bililiuliangfa18_4) -> SQfa/3(bililiuliangfa18_4)
  p1sheding/1 -> Chart/8(p1sheding)
  p0sheding/1 -> Chart/13(p0sheding)
  p0_0/1 -> Chart/12(p0_0)
  p2/1 -> Chart/10(p2), [p2]
  p3/1 -> Chart/11(p3), [p3]
  [p3] -> XQfa/1(p3)
  [p2] -> SQfa/1(p2)
  p1/1 -> Chart/7(p1)
  start/1 -> Chart/1(start)
  Chart/1(diancifa11_1) -> diancifa11_1/1
  SCzhushui/1 -> Chart/2(SCzhushui)
  Chart/2(diancifa11_2) -> diancifa11_2/1
  fuqiuyeweikongzhiqi/1 -> Chart/3(fuqiuyeweikongzhiqi)
  Chart/3(diancifa11_5) -> diancifa11_5/1
  SCjiaya/1 -> Chart/4(SCjiaya)
  Chart/4(diancifa20) -> diancifa20/1
  SXQjunya/1 -> Chart/5(SXQjunya)
  Chart/5(diancifa16_1) -> diancifa16_1/1
  SXQxieya/1 -> Chart/6(SXQxieya)
  Chart/6(diancifa3) -> diancifa3/1
  XQfa/1(fa18_1) -> bililiuliangfa18_1/1
  Chart/7(diancifa21) -> diancifa21/1
  XQfa/2(fa18_3) -> bililiuliangfa18_3/1
  liuliangji/1 -> Chart/9(liuliangji)
  SQfa/1(fa18_2) -> bililiuliangfa18_2/1
  SQfa/2(fa18_4) -> bililiuliangfa18_4/1
  zidongkaigai/1 -> Chart/25(zidongkaigai)
  zidongguangai/1 -> Chart/26(zidongguangai)
  xuansongdaowei1/1 -> Chart/14(xuansongdaowei1)
  xuansongdaowei2/1 -> Chart/15(xuansongdaowei2)
  xuanjindaowei1/1 -> Chart/16(xuanjindaowei1)
  xuanjindaowei2/1 -> Chart/17(xuanjindaowei2)
  suodingdaowei1/1 -> Chart/18(suodingdaowei1)
  suodingdaowei2/1 -> Chart/19(suodingdaowei2)
  jiesuodaowei1/1 -> Chart/20(jiesuodaowei1)
  jiesuodaowei2/1 -> Chart/21(jiesuodaowei2)
  kaigaijieshu/1 -> Chart/22(kaigaijieshu)
  Chart/24(kaigaiwancheng) -> kaigaiwancheng/1
  guangaijieshu/1 -> Chart/23(guangaijieshu)
  Chart/25(guangaiwancheng) -> guangaiwancheng/1
  Chart/8(suoding) -> dianyehuanxiangfa42_1/1
  Chart/9(jiesuo) -> dianyehuanxiangfa42_2/1
  Chart/18(SCzhushuiwancheng) -> SCzhushuiwancheng/1
  Chart/19(SCjiayawancheng) -> SCjiayawancheng/1
  Chart/20(SXQjunyawancheng) -> SXQjunyawancheng/1
  Chart/21(SXQxieyawancheng) -> SXQxieyawancheng/1
  Chart/22(SQshiyabuchangwancheng) -> SQshiyabuchangwancheng/1
  Chart/23(SQxuanjinjianyawancheng) -> SQxuanjinjianyawancheng/1
  xkgg/1 -> [xkgg]
  jiting/1 -> Chart/24(jiting)
  xxsj1/1 -> [xxsj1]
  xxsj2/1 -> [xxsj2]
  Chart/16(kaigaikaishi) -> kaigaikaishi/1, Subsystem/1(kaigaikaishi)
  Chart/17(guangaikaishi) -> guangaikaishi/1, Subsystem/2(guangaikaishi)
  [xkgg] -> Subsystem/5(xkgg)
  Subsystem/1(Out1) -> kaiguangaifa/1
  [xxsj2] -> Subsystem1/4(xxsj2)
  [xxsj1] -> Subsystem1/3(xxsj1)
  Chart/10(xuansong) -> xuansong/1
  Chart/11(xuanjin) -> xuanjin/1
  kaigaiquxian/1 -> Subsystem/3(kaigaiquxian)
  guangaiquxian/1 -> Subsystem/4(guangaiquxian)

== system aaaqi/chuanganqi/yalishangxiaxian ==
  In1 : Inport
  Compare To Constant{1,3,5,7,9,11} (6 alike) : simulink/Logic and Bit Operations/Compare To Constant  relop=>=  const=0.33  OutDataTypeStr=boolean
  Demux5 : Demux  Outputs=6
  Logical Operator : Logic  Operator=OR  Inputs=6  AllPortsSameDT=off  OutDataTypeStr=boolean
  Out1 : Outport
  wires:
  Demux5/2 -> Compare To Constant3/1
  Demux5/6 -> Compare To Constant11/1
  Demux5/4 -> Compare To Constant7/1
  Demux5/3 -> Compare To Constant5/1
  Demux5/1 -> Compare To Constant1/1
  Demux5/5 -> Compare To Constant9/1
  In1/1 -> Demux5/1
  Logical Operator/1 -> Out1/1
  Compare To Constant11/1 -> Logical Operator/6
  Compare To Constant9/1 -> Logical Operator/5
  Compare To Constant7/1 -> Logical Operator/4
  Compare To Constant5/1 -> Logical Operator/3
  Compare To Constant3/1 -> Logical Operator/2
  Compare To Constant1/1 -> Logical Operator/1

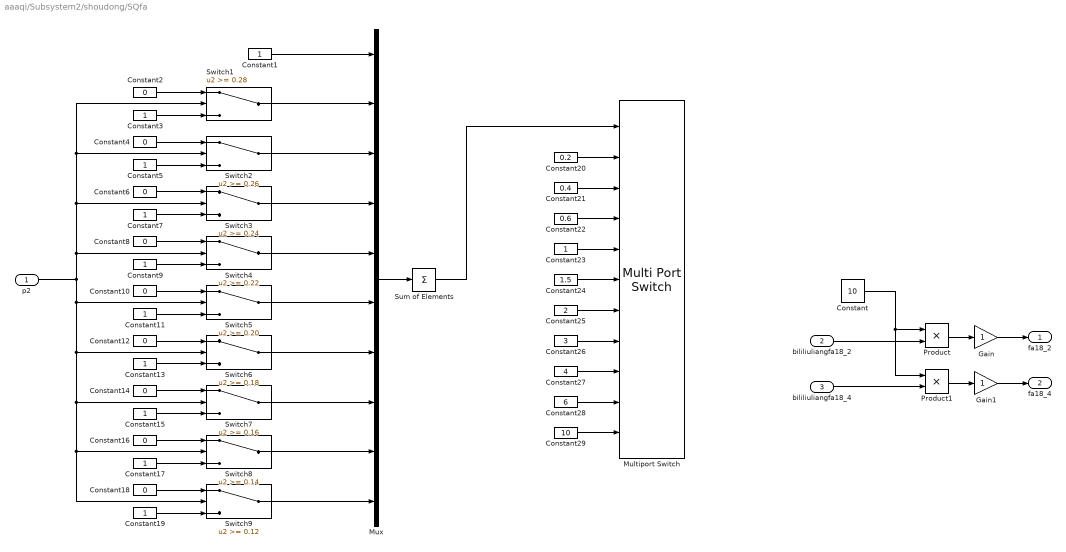
== system aaaqi/Subsystem2/shoudong/SQfa ==
  p2 : Inport
  bililiuliangfa18_2 : Inport  Port=2
  bililiuliangfa18_4 : Inport  Port=3
  Constant : Constant  Value=10
  Constant{1,3,5,7,9,11,13,15,17,19,23} (11 alike) : Constant
  Constant{2,4,6,8,10,12,14,16,18} (9 alike) : Constant  Value=0
  Constant20 : Constant  Value=0.2
  Constant21 : Constant  Value=0.4
  Constant22 : Constant  Value=0.6
  Constant24 : Constant  Value=1.5
  Constant25 : Constant  Value=2
  Constant26 : Constant  Value=3
  Constant27 : Constant  Value=4
  Constant28 : Constant  Value=6
  Constant29 : Constant  Value=10
  Gain : Gain
  Gain1 : Gain
  Multiport Switch : MultiPortSwitch  Inputs=10
  Mux : Mux  Inputs=10
  Product : Product  RndMeth=Zero
  Product1 : Product  RndMeth=Zero
  Sum of Elements : Sum  Inputs=+
  Switch1 : Switch  Threshold=0.28
  Switch2 : Switch  Threshold=0.26
  Switch3 : Switch  Threshold=0.24
  Switch4 : Switch  Threshold=0.22
  Switch5 : Switch  Threshold=0.20
  Switch6 : Switch  Threshold=0.18
  Switch7 : Switch  Threshold=0.16
  Switch8 : Switch  Threshold=0.14
  Switch9 : Switch  Threshold=0.12
  fa18_2 : Outport
  fa18_4 : Outport  Port=2
  wires:
  Constant2/1 -> Switch1/1
  Constant3/1 -> Switch1/3
  Constant4/1 -> Switch2/1
  Constant5/1 -> Switch2/3
  Constant6/1 -> Switch3/1
  Constant7/1 -> Switch3/3
  Constant8/1 -> Switch4/1
  Constant9/1 -> Switch4/3
  Constant10/1 -> Switch5/1
  Constant11/1 -> Switch5/3
  Constant12/1 -> Switch6/1
  Constant13/1 -> Switch6/3
  Constant14/1 -> Switch7/1
  Constant15/1 -> Switch7/3
  p2/1 -> Switch1/2, Switch2/2, Switch3/2, Switch4/2, Switch6/2, Switch7/2, Switch8/2, Switch9/2, Switch5/2
  Mux/1 -> Sum of Elements/1
  Sum of Elements/1 -> Multiport Switch/1
  Constant1/1 -> Mux/1
  Switch1/1 -> Mux/2
  Switch2/1 -> Mux/3
  Switch3/1 -> Mux/4
  Switch4/1 -> Mux/5
  Switch5/1 -> Mux/6
  Switch6/1 -> Mux/7
  Switch7/1 -> Mux/8
  Switch8/1 -> Mux/9
  Switch9/1 -> Mux/10
  Constant16/1 -> Switch8/1
  Constant17/1 -> Switch8/3
  Constant18/1 -> Switch9/1
  Constant19/1 -> Switch9/3
  Constant20/1 -> Multiport Switch/2
  Constant21/1 -> Multiport Switch/3
  Constant22/1 -> Multiport Switch/4
  Constant23/1 -> Multiport Switch/5
  Constant24/1 -> Multiport Switch/6
  Constant25/1 -> Multiport Switch/7
  Constant26/1 -> Multiport Switch/8
  Constant27/1 -> Multiport Switch/9
  Constant28/1 -> Multiport Switch/10
  Constant29/1 -> Multiport Switch/11
  bililiuliangfa18_2/1 -> Product/2
  bililiuliangfa18_4/1 -> Product1/2
  Product/1 -> Gain/1
  Product1/1 -> Gain1/1
  Gain/1 -> fa18_2/1
  Gain1/1 -> fa18_4/1
  Constant/1 -> Product1/1, Product/1

== system aaaqi/Subsystem2/shoudong/Subsystem ==
  kaigaikaishi : Inport
  guangaikaishi : Inport  Port=2
  kaigaiquxian : Inport  Port=3
  guangaiquxian : Inport  Port=4
  xkgg : Inport  Port=5
  Add1 : Sum
  Constant : Constant  Value=2
  Constant1 : Constant  Value=-0.05
  Display{,1..3} (4 alike) : Display
  Gain : Gain  Gain=0.15
  Gain1 : Gain  Gain=0.15
  Multiport Switch : MultiPortSwitch
  Product : Product
  Sum : Sum  Inputs=|+-
  Sum1 : Sum  Inputs=|+-
  Out1 : Outport
  wires:
  guangaikaishi/1 -> Product/1
  Constant/1 -> Product/2
  kaigaikaishi/1 -> Add1/1
  Product/1 -> Add1/2
  Add1/1 -> Multiport Switch/1
  Multiport Switch/1 -> Display2/1, Out1/1
  Sum/1 -> Gain/1
  Gain/1 -> Multiport Switch/2, Display1/1
  Sum1/1 -> Gain1/1
  Gain1/1 -> Display/1, Multiport Switch/3
  Constant1/1 -> Multiport Switch/4
  xkgg/1 -> Display3/1, Sum1/2, Sum/2
  kaigaiquxian/1 -> Sum/1
  guangaiquxian/1 -> Sum1/1

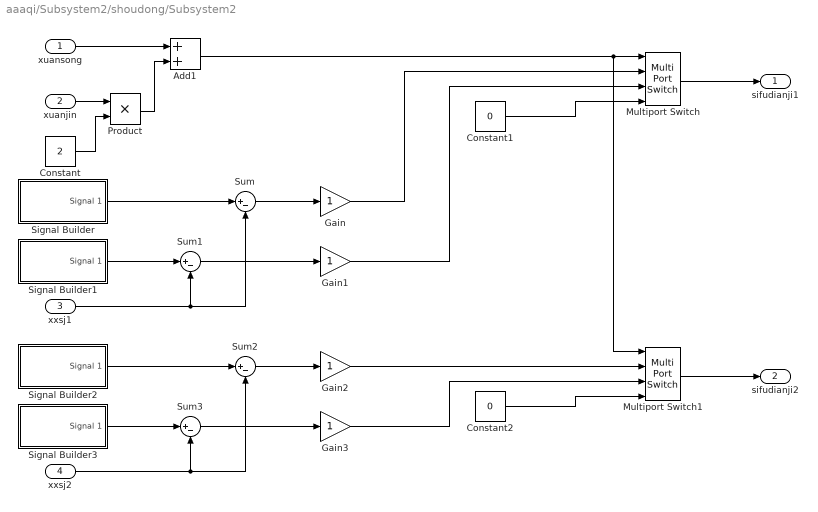
== system aaaqi/Subsystem2/shoudong/Subsystem2 ==
  xuansong : Inport
  xuanjin : Inport  Port=2
  xxsj1 : Inport  Port=3
  xxsj2 : Inport  Port=4
  Add1 : Sum
  Constant : Constant  Value=2
  Constant1 : Constant  Value=0
  Constant2 : Constant  Value=0
  Gain{,1..3} (4 alike) : Gain
  Multiport Switch : MultiPortSwitch
  Multiport Switch1 : MultiPortSwitch
  Product : Product
  Signal Builder : Subsystem  Tag=STV Subsys  LoadFcn=sigbuilder_block('load');  StartFcn=sigbuilder_block('start');  StopFcn=sigbuilder_block('stop');  ClipboardFcn=sigbuilder_block('clipboard');  mask(Sigbuilder block){tuvar=[0:10]}
      mask help: Simulink:masks:SigbuilderBlock_MD
      mask init:
      | if ~strcmp(get_param(bdroot(gcbh),'SimulationStatus'),'stopped') tuvar = sigbuilder_block('maskInit'); end
      settings: CopyFcn=sigbuilder_block('copy');  DeleteFcn=sigbuilder_block('delete');  ModelCloseFcn=sigbuilder_block('modelClose');  PreSaveFcn=sigbuilder_block('preSave');  PauseFcn=sigbuilder_block('pause');  ContinueFcn=sigbuilder_block('continue');  NameChangeFcn=sigbuilder_block('namechange');  OpenFcn=sigbuilder_block('open',[437.6 199.2 550.4 400 ]);  CloseFcn=sigbuilder_block('close');
      mask Display: plot(0, 0, 100, 100,[2, 2, 32, 32, 2], [68, 8, 8, 68, 68],[32, 2], [38, 38], [32, 19, 2],[53, 60, 44], [32, 17, 17, 2],[16, 16, 31, 31]);txt = getActiveGroup(gcbh);text(2, 100, txt,'verticalAlignment', 'top');
  Signal Builder1 : Subsystem  Tag=STV Subsys  LoadFcn=sigbuilder_block('load');  StartFcn=sigbuilder_block('start');  StopFcn=sigbuilder_block('stop');  ClipboardFcn=sigbuilder_block('clipboard');  mask(Sigbuilder block){tuvar=[0:10]}
      mask help: Simulink:masks:SigbuilderBlock_MD
      mask init:
      | if ~strcmp(get_param(bdroot(gcbh),'SimulationStatus'),'stopped') tuvar = sigbuilder_block('maskInit'); end
      settings: CopyFcn=sigbuilder_block('copy');  DeleteFcn=sigbuilder_block('delete');  ModelCloseFcn=sigbuilder_block('modelClose');  PreSaveFcn=sigbuilder_block('preSave');  PauseFcn=sigbuilder_block('pause');  ContinueFcn=sigbuilder_block('continue');  NameChangeFcn=sigbuilder_block('namechange');  OpenFcn=sigbuilder_block('open',[437.6 199.2 550.4 400 ]);  CloseFcn=sigbuilder_block('close');
      mask Display: plot(0, 0, 100, 100,[2, 2, 32, 32, 2], [68, 8, 8, 68, 68],[32, 2], [38, 38], [32, 19, 2],[53, 60, 44], [32, 17, 17, 2],[16, 16, 31, 31]);txt = getActiveGroup(gcbh);text(2, 100, txt,'verticalAlignment', 'top');
  Signal Builder2 : Subsystem  Tag=STV Subsys  LoadFcn=sigbuilder_block('load');  StartFcn=sigbuilder_block('start');  StopFcn=sigbuilder_block('stop');  ClipboardFcn=sigbuilder_block('clipboard');  mask(Sigbuilder block){tuvar=[0:10]}
      mask help: Simulink:masks:SigbuilderBlock_MD
      mask init:
      | if ~strcmp(get_param(bdroot(gcbh),'SimulationStatus'),'stopped') tuvar = sigbuilder_block('maskInit'); end
      settings: CopyFcn=sigbuilder_block('copy');  DeleteFcn=sigbuilder_block('delete');  ModelCloseFcn=sigbuilder_block('modelClose');  PreSaveFcn=sigbuilder_block('preSave');  PauseFcn=sigbuilder_block('pause');  ContinueFcn=sigbuilder_block('continue');  NameChangeFcn=sigbuilder_block('namechange');  OpenFcn=sigbuilder_block('open',[437.6 199.2 550.4 400 ]);  CloseFcn=sigbuilder_block('close');
      mask Display: plot(0, 0, 100, 100,[2, 2, 32, 32, 2], [68, 8, 8, 68, 68],[32, 2], [38, 38], [32, 19, 2],[53, 60, 44], [32, 17, 17, 2],[16, 16, 31, 31]);txt = getActiveGroup(gcbh);text(2, 100, txt,'verticalAlignment', 'top');
  Signal Builder3 : Subsystem  Tag=STV Subsys  LoadFcn=sigbuilder_block('load');  StartFcn=sigbuilder_block('start');  StopFcn=sigbuilder_block('stop');  ClipboardFcn=sigbuilder_block('clipboard');  mask(Sigbuilder block){tuvar=[0:10]}
      mask help: Simulink:masks:SigbuilderBlock_MD
      mask init:
      | if ~strcmp(get_param(bdroot(gcbh),'SimulationStatus'),'stopped') tuvar = sigbuilder_block('maskInit'); end
      settings: CopyFcn=sigbuilder_block('copy');  DeleteFcn=sigbuilder_block('delete');  ModelCloseFcn=sigbuilder_block('modelClose');  PreSaveFcn=sigbuilder_block('preSave');  PauseFcn=sigbuilder_block('pause');  ContinueFcn=sigbuilder_block('continue');  NameChangeFcn=sigbuilder_block('namechange');  OpenFcn=sigbuilder_block('open',[437.6 199.2 550.4 400 ]);  CloseFcn=sigbuilder_block('close');
      mask Display: plot(0, 0, 100, 100,[2, 2, 32, 32, 2], [68, 8, 8, 68, 68],[32, 2], [38, 38], [32, 19, 2],[53, 60, 44], [32, 17, 17, 2],[16, 16, 31, 31]);txt = getActiveGroup(gcbh);text(2, 100, txt,'verticalAlignment', 'top');
  Sum{,1..3} (4 alike) : Sum  Inputs=|+-
  sifudianji1 : Outport
  sifudianji2 : Outport  Port=2
  wires:
  Constant1/1 -> Multiport Switch/4
  Gain1/1 -> Multiport Switch/3
  Sum1/1 -> Gain1/1
  Signal Builder1/1(Signal 1) -> Sum1/1
  Gain/1 -> Multiport Switch/2
  Sum/1 -> Gain/1
  xxsj1/1 -> Sum/2, Sum1/2
  Signal Builder/1(Signal 1) -> Sum/1
  Multiport Switch/1 -> sifudianji1/1
  Add1/1 -> Multiport Switch1/1, Multiport Switch/1
  Product/1 -> Add1/2
  xuansong/1 -> Add1/1
  Constant/1 -> Product/2
  xuanjin/1 -> Product/1
  Multiport Switch1/1 -> sifudianji2/1
  Signal Builder2/1(Signal 1) -> Sum2/1
  xxsj2/1 -> Sum2/2, Sum3/2
  Sum2/1 -> Gain2/1
  Gain2/1 -> Multiport Switch1/2
  Signal Builder3/1(Signal 1) -> Sum3/1
  Sum3/1 -> Gain3/1
  Gain3/1 -> Multiport Switch1/3
  Constant2/1 -> Multiport Switch1/4

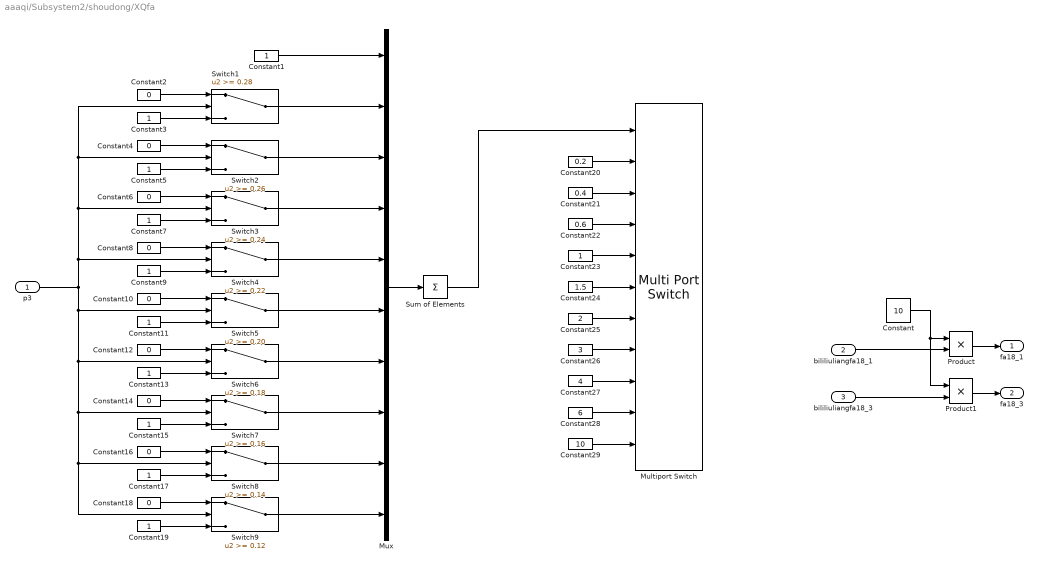
== system aaaqi/Subsystem2/shoudong/XQfa ==
  p3 : Inport
  bililiuliangfa18_1 : Inport  Port=2
  bililiuliangfa18_3 : Inport  Port=3
  Constant : Constant  Value=10
  Constant{1,3,5,7,9,11,13,15,17,19,23} (11 alike) : Constant
  Constant{2,4,6,8,10,12,14,16,18} (9 alike) : Constant  Value=0
  Constant20 : Constant  Value=0.2
  Constant21 : Constant  Value=0.4
  Constant22 : Constant  Value=0.6
  Constant24 : Constant  Value=1.5
  Constant25 : Constant  Value=2
  Constant26 : Constant  Value=3
  Constant27 : Constant  Value=4
  Constant28 : Constant  Value=6
  Constant29 : Constant  Value=10
  Multiport Switch : MultiPortSwitch  Inputs=10
  Mux : Mux  Inputs=10
  Product : Product  RndMeth=Zero
  Product1 : Product  RndMeth=Zero
  Sum of Elements : Sum  Inputs=+
  Switch1 : Switch  Threshold=0.28
  Switch2 : Switch  Threshold=0.26
  Switch3 : Switch  Threshold=0.24
  Switch4 : Switch  Threshold=0.22
  Switch5 : Switch  Threshold=0.20
  Switch6 : Switch  Threshold=0.18
  Switch7 : Switch  Threshold=0.16
  Switch8 : Switch  Threshold=0.14
  Switch9 : Switch  Threshold=0.12
  fa18_1 : Outport
  fa18_3 : Outport  Port=2
  wires:
  Product1/1 -> fa18_3/1
  Product/1 -> fa18_1/1
  bililiuliangfa18_3/1 -> Product1/2
  bililiuliangfa18_1/1 -> Product/2
  Constant29/1 -> Multiport Switch/11
  Constant28/1 -> Multiport Switch/10
  Constant27/1 -> Multiport Switch/9
  Constant26/1 -> Multiport Switch/8
  Constant25/1 -> Multiport Switch/7
  Constant24/1 -> Multiport Switch/6
  Constant23/1 -> Multiport Switch/5
  Constant22/1 -> Multiport Switch/4
  Constant21/1 -> Multiport Switch/3
  Constant20/1 -> Multiport Switch/2
  Constant19/1 -> Switch9/3
  Constant18/1 -> Switch9/1
  Constant17/1 -> Switch8/3
  Constant16/1 -> Switch8/1
  Switch9/1 -> Mux/10
  Switch8/1 -> Mux/9
  Switch7/1 -> Mux/8
  Switch6/1 -> Mux/7
  Switch5/1 -> Mux/6
  Switch4/1 -> Mux/5
  Switch3/1 -> Mux/4
  Switch2/1 -> Mux/3
  Switch1/1 -> Mux/2
  Constant1/1 -> Mux/1
  Sum of Elements/1 -> Multiport Switch/1
  Mux/1 -> Sum of Elements/1
  p3/1 -> Switch5/2, Switch9/2, Switch8/2, Switch7/2, Switch6/2, Switch4/2, Switch3/2, Switch2/2, Switch1/2
  Constant15/1 -> Switch7/3
  Constant14/1 -> Switch7/1
  Constant13/1 -> Switch6/3
  Constant12/1 -> Switch6/1
  Constant11/1 -> Switch5/3
  Constant10/1 -> Switch5/1
  Constant9/1 -> Switch4/3
  Constant8/1 -> Switch4/1
  Constant7/1 -> Switch3/3
  Constant6/1 -> Switch3/1
  Constant5/1 -> Switch2/3
  Constant4/1 -> Switch2/1
  Constant3/1 -> Switch1/3
  Constant2/1 -> Switch1/1
  Constant/1 -> Product1/1, Product/1

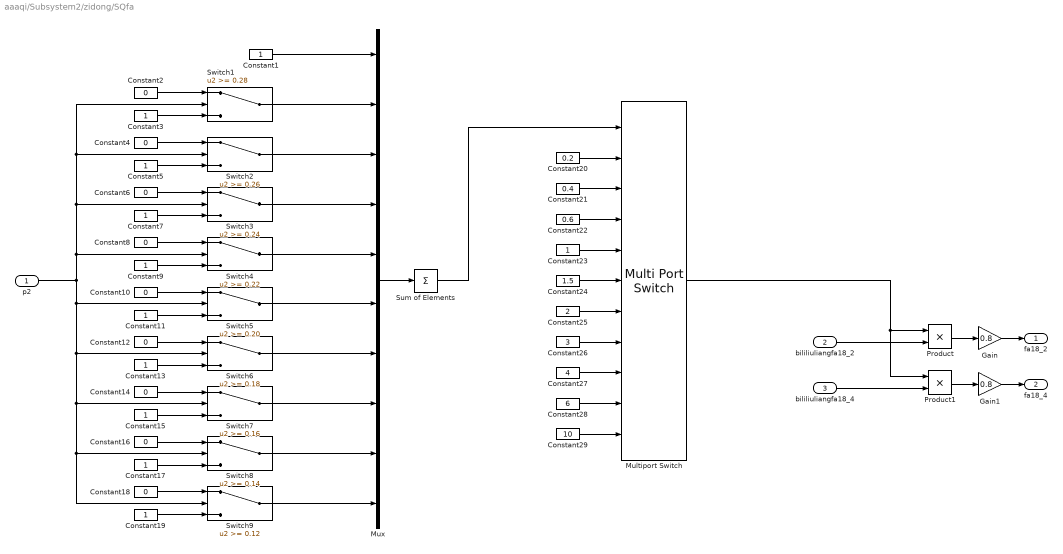
== system aaaqi/Subsystem2/zidong/SQfa ==
  p2 : Inport
  bililiuliangfa18_2 : Inport  Port=2
  bililiuliangfa18_4 : Inport  Port=3
  Constant{1,3,5,7,9,11,13,15,17,19,23} (11 alike) : Constant
  Constant{2,4,6,8,10,12,14,16,18} (9 alike) : Constant  Value=0
  Constant20 : Constant  Value=0.2
  Constant21 : Constant  Value=0.4
  Constant22 : Constant  Value=0.6
  Constant24 : Constant  Value=1.5
  Constant25 : Constant  Value=2
  Constant26 : Constant  Value=3
  Constant27 : Constant  Value=4
  Constant28 : Constant  Value=6
  Constant29 : Constant  Value=10
  Gain : Gain  Gain=0.8
  Gain1 : Gain  Gain=0.8
  Multiport Switch : MultiPortSwitch  Inputs=10
  Mux : Mux  Inputs=10
  Product : Product  RndMeth=Zero
  Product1 : Product  RndMeth=Zero
  Sum of Elements : Sum  Inputs=+
  Switch1 : Switch  Threshold=0.28
  Switch2 : Switch  Threshold=0.26
  Switch3 : Switch  Threshold=0.24
  Switch4 : Switch  Threshold=0.22
  Switch5 : Switch  Threshold=0.20
  Switch6 : Switch  Threshold=0.18
  Switch7 : Switch  Threshold=0.16
  Switch8 : Switch  Threshold=0.14
  Switch9 : Switch  Threshold=0.12
  fa18_2 : Outport
  fa18_4 : Outport  Port=2
  wires:
  Product1/1 -> Gain1/1
  Product/1 -> Gain/1
  bililiuliangfa18_4/1 -> Product1/2
  bililiuliangfa18_2/1 -> Product/2
  Constant29/1 -> Multiport Switch/11
  Constant28/1 -> Multiport Switch/10
  Constant27/1 -> Multiport Switch/9
  Constant26/1 -> Multiport Switch/8
  Constant25/1 -> Multiport Switch/7
  Constant24/1 -> Multiport Switch/6
  Constant23/1 -> Multiport Switch/5
  Constant22/1 -> Multiport Switch/4
  Constant21/1 -> Multiport Switch/3
  Constant20/1 -> Multiport Switch/2
  Multiport Switch/1 -> Product1/1, Product/1
  Constant19/1 -> Switch9/3
  Constant18/1 -> Switch9/1
  Constant17/1 -> Switch8/3
  Constant16/1 -> Switch8/1
  Switch9/1 -> Mux/10
  Switch8/1 -> Mux/9
  Switch7/1 -> Mux/8
  Switch6/1 -> Mux/7
  Switch5/1 -> Mux/6
  Switch4/1 -> Mux/5
  Switch3/1 -> Mux/4
  Switch2/1 -> Mux/3
  Switch1/1 -> Mux/2
  Constant1/1 -> Mux/1
  Sum of Elements/1 -> Multiport Switch/1
  Mux/1 -> Sum of Elements/1
  p2/1 -> Switch5/2, Switch9/2, Switch8/2, Switch7/2, Switch6/2, Switch4/2, Switch3/2, Switch2/2, Switch1/2
  Constant15/1 -> Switch7/3
  Constant14/1 -> Switch7/1
  Constant13/1 -> Switch6/3
  Constant12/1 -> Switch6/1
  Constant11/1 -> Switch5/3
  Constant10/1 -> Switch5/1
  Constant9/1 -> Switch4/3
  Constant8/1 -> Switch4/1
  Constant7/1 -> Switch3/3
  Constant6/1 -> Switch3/1
  Constant5/1 -> Switch2/3
  Constant4/1 -> Switch2/1
  Constant3/1 -> Switch1/3
  Constant2/1 -> Switch1/1
  Gain/1 -> fa18_2/1
  Gain1/1 -> fa18_4/1
